simulink model "mdl_tubing_simevents"  (R2020b)
settings: Solver=VariableStepAuto  StartTime=0.0  StopTime=100.0  RelTol=1e-3
undefined symbols (not defined in the file): m, n
settings Model: Creator=natha  LastModifiedBy=natha

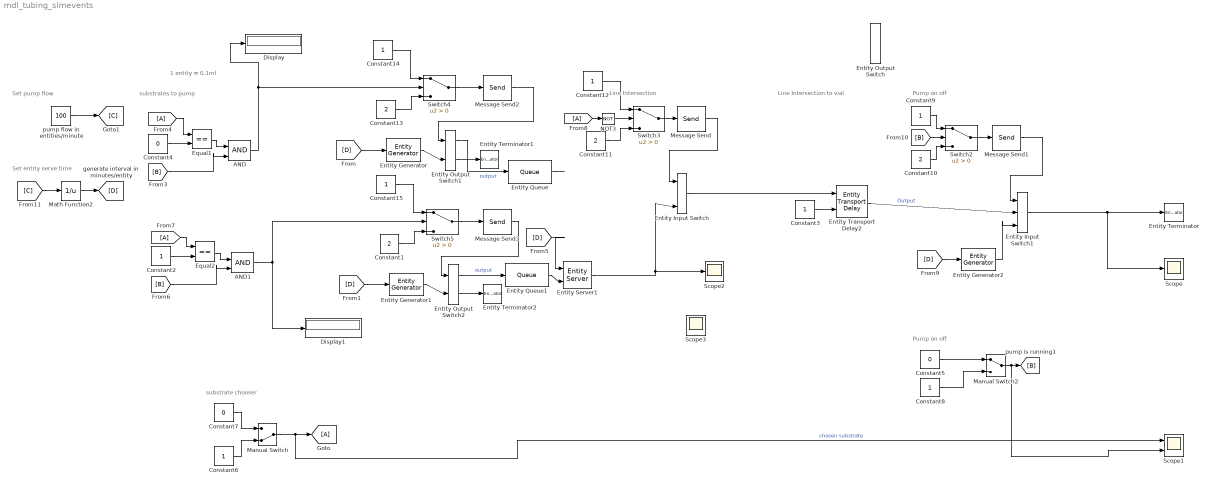
== system mdl_tubing_simevents ==
  note: Pump on off
  note: Line Intersection to vial
  note: Set pump flow
  note: 1 entity = 0.1ml
  note: substrate chooser
  note: substrates to pump
  note: Pump on off
  note: Line Intersection
  note: Set entity serve time
  AND : Logic  IconShape=distinctive  AllPortsSameDT=off  OutDataTypeStr=boolean
  AND1 : Logic  IconShape=distinctive  AllPortsSameDT=off  OutDataTypeStr=boolean
  Constant{1,10..11,13} (4 alike) : Constant  Value=2
  Constant{2..3,6,8..9,12,14..15} (8 alike) : Constant
  Constant4 : Constant  Value=0
  Constant5 : Constant  Value=0
  Constant7 : Constant  Value=0
  Display : Display
  Display1 : Display
  Entity Input Switch : EntityInputSwitch  InputPortMessageModes=m,m,m  OutputPortMessageModes=m  ActivePortSelection=Switch  SwitchingCriterion=From control port
      settings: InputPortMap=u0,u1,u2
  Entity Input Switch1 : EntityInputSwitch  InputPortMessageModes=m,m,m  OutputPortMessageModes=m  ActivePortSelection=Switch  SwitchingCriterion=From control port
      settings: InputPortMap=u0,u1,u2
  Entity Output Switch : EntityOutputSwitch  InputPortMessageModes=m  OutputPortMessageModes=m,m  SwitchAttributeName=Attribute1
  Entity Output Switch1 : EntityOutputSwitch  InputPortMessageModes=m,m  OutputPortMessageModes=m,m  SwitchingCriterion=From control port  SwitchAttributeName=Attribute1
      settings: InputPortMap=u0,u1
  Entity Output Switch2 : EntityOutputSwitch  InputPortMessageModes=m,m  OutputPortMessageModes=m,m  SwitchingCriterion=From control port  SwitchAttributeName=Attribute1
      settings: InputPortMap=u0,u1
  Entity Transport Delay2 : EntityTransportDelay  InputPortMessageModes=m,n  OutputPortMessageModes=m
  Entity Generator : EntityGenerator  OutputPortMessageModes=m  TimeSource=Signal port  GenerateEntityAtSimulationStart=off  AttributeName=Substrate  AttributeInitialValue=0  EntityType=Structured  EntityTypeName=Entity
      settings: InputPortMap=u1
  Entity Generator1 : EntityGenerator  OutputPortMessageModes=m  TimeSource=Signal port  GenerateEntityAtSimulationStart=off  AttributeName=Substrate  AttributeInitialValue=0  EntityType=Structured  EntityTypeName=Entity
      settings: InputPortMap=u1
  Entity Generator2 : EntityGenerator  OutputPortMessageModes=m  TimeSource=Signal port  GenerateEntityAtSimulationStart=off  AttributeName=Substrate  AttributeInitialValue=-1  EntityType=Structured  EntityTypeName=Entity
      settings: InputPortMap=u1
  Entity Queue : Queue  InputPortMessageModes=m  OutputPortMessageModes=m
  Entity Queue1 : Queue  InputPortMessageModes=m  OutputPortMessageModes=m
  Entity Server1 : EntityServer  InputPortMessageModes=n,m  OutputPortMessageModes=m  Capacity=1  ServiceTimeSource=Signal port
      settings: InputPortMap=u0,u2
  Entity Terminator : EntityTerminator  InputPortMessageModes=m
  Entity Terminator1 : EntityTerminator  InputPortMessageModes=m
  Entity Terminator2 : EntityTerminator  InputPortMessageModes=m
  Equal1 : RelationalOperator  Operator===  OutDataTypeStr=boolean  RndMeth=Simplest
  Equal2 : RelationalOperator  Operator===  OutDataTypeStr=boolean  RndMeth=Simplest
  Manual Switch : ManualSwitch  CurrentSetting=0
  Manual Switch2 : ManualSwitch
  Math Function2 : Math  Operator=reciprocal  SaturateOnIntegerOverflow=on
  Message Send{,1..3} (4 alike) : Send  OutputPortMessageModes=m
  NOT3 : Logic  Operator=NOT  IconShape=distinctive  AllPortsSameDT=off  OutDataTypeStr=boolean
  Scope : Scope
  Scope1 : Scope  NumInputPorts=2
  Scope2 : Scope
  Scope3 : Scope
  Switch{2..5} (4 alike) : Switch  Criteria=u2 > Threshold
  pump flow in entities/minute : Constant  Value=100
  wires:
  Constant4/1 -> Equal1/2
  Equal1/1 -> AND/1
  [B] -> AND/2
  [A] -> Equal1/1
  Manual Switch/1 -> Scope1/1, [A]  "chosen substrate"
  Constant6/1 -> Manual Switch/2
  Constant7/1 -> Manual Switch/1
  AND/1 -> Switch4/2, Display/1
  pump flow in entities/minute/1 -> [C]
  [A] -> Equal2/1
  [B] -> AND1/2
  Equal2/1 -> AND1/1
  Constant2/1 -> Equal2/2
  Entity Transport Delay2/1 -> Entity Input Switch1/2  "Output"
  Entity Input Switch/1 -> Entity Transport Delay2/1
  Entity Output Switch2/1 -> Entity Queue1/1  "output"
  Entity Output Switch1/1 -> Entity Queue/1  "output"
  Constant3/1 -> Entity Transport Delay2/2
  Entity Generator2/1 -> Entity Input Switch1/3
  [D] -> Entity Generator2/1
  Manual Switch2/1 -> Scope1/2, [B]
  Constant5/1 -> Manual Switch2/1
  Constant8/1 -> Manual Switch2/2
  Entity Input Switch1/1 -> Scope/1, Entity Terminator/1
  [A] -> NOT3/1
  Message Send/1 -> Entity Input Switch/1
  [B] -> Switch2/2
  Message Send1/1 -> Entity Input Switch1/1
  Switch2/1 -> Message Send1/1
  Constant9/1 -> Switch2/1
  Constant10/1 -> Switch2/3
  Constant11/1 -> Switch3/3
  Constant12/1 -> Switch3/1
  Switch3/1 -> Message Send/1
  NOT3/1 -> Switch3/2
  Math Function2/1 -> [D]
  [C] -> Math Function2/1
  Entity Generator/1 -> Entity Output Switch1/2
  [D] -> Entity Generator/1
  Constant14/1 -> Switch4/1
  Constant13/1 -> Switch4/3
  Message Send2/1 -> Entity Output Switch1/1
  Entity Output Switch1/2 -> Entity Terminator1/1
  Entity Output Switch2/2 -> Entity Terminator2/1
  Constant15/1 -> Switch5/1
  Entity Generator1/1 -> Entity Output Switch2/2
  [D] -> Entity Generator1/1
  Constant1/1 -> Switch5/3
  Message Send3/1 -> Entity Output Switch2/1
  AND1/1 -> Switch5/2, Display1/1
  Switch4/1 -> Message Send2/1
  Switch5/1 -> Message Send3/1
  ? -> Scope3/1, Entity Input Switch/2
  Entity Server1/1 -> Entity Input Switch/3, Scope2/1
  [D] -> Entity Server1/1
  Entity Queue/1 -> ?
  Entity Queue1/1 -> Entity Server1/2
